simulink model "hydrothermal"  (R2018b)
settings: Solver=ode45  StartTime=0.0  StopTime=100  FixedStep=2  RelTol=1e-3
values from neighbouring files (symbols this model uses):
  optim_param = Best_pos    [main.m]
  w1 = 0.001    [main.m]
  w2 = 0.001    [main.m]
libraries: powerlib x1
settings Model: Creator=Orka  LastModifiedBy=Orka
settings SolverCC: ZeroCrossAlgorithm=Adaptive
settings DataIOCC: Refine=10
settings DebuggingCC: MaskedZcDiagnostic=none  IgnoredZcDiagnostic=none

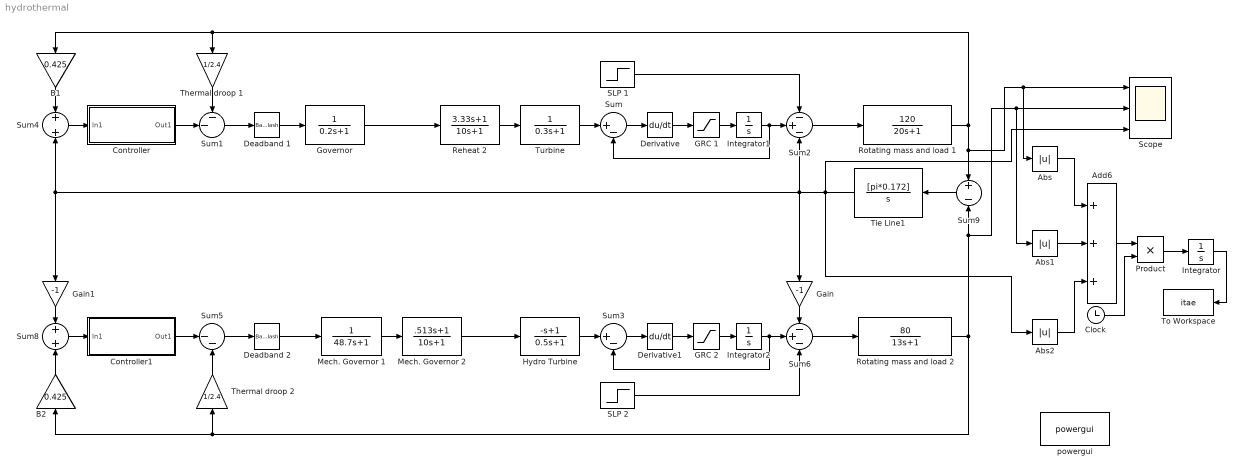
== system hydrothermal ==
  Abs : Abs
  Abs1 : Abs
  Abs2 : Abs
  Add6 : Sum  Inputs=+++
  B1 : Gain  Gain=0.425
  B2 : Gain  Gain=0.425
  Clock : Clock
  Controller : Subsystem
  Controller1 : Subsystem
  Deadband 1 : Backlash  BacklashWidth=0.0005
  Deadband 2 : Backlash  BacklashWidth=0.0002
  Derivative : Derivative
  Derivative1 : Derivative
  GRC 1 : Saturate  UpperLimit=0.0017  LowerLimit=-0.0017
  GRC 2 : Saturate  UpperLimit=0.045  LowerLimit=-0.06
  Gain : Gain  Gain=-1
  Gain1 : Gain  Gain=-1
  Governor : TransferFcn  Denominator=[0.2 1]
  Hydro Turbine : TransferFcn  Numerator=[-1 1]  Denominator=[0.5 1]
  Integrator : Integrator
  Integrator1 : Integrator
  Integrator2 : Integrator
  Mech. Governor 1 : TransferFcn  Denominator=[48.7 1]
  Mech. Governor 2 : TransferFcn  Numerator=[.513 1]  Denominator=[10 1]
  Product : Product
  Reheat 2 : TransferFcn  Numerator=[3.33 1]  Denominator=[10 1]
  Rotating mass and load 1 : TransferFcn  Numerator=[120]  Denominator=[20 1]
  Rotating mass and load 2 : TransferFcn  Numerator=[80]  Denominator=[13 1]
  SLP 1 : Step  After=w1  SampleTime=0
  SLP 2 : Step  After=w2  SampleTime=0
  Scope : Scope  NumInputPorts=3
  Sum : Sum  Inputs=|+-
  Sum1 : Sum  Inputs=--|
  Sum2 : Sum  Inputs=-+-
  Sum3 : Sum  Inputs=|+-
  Sum4 : Sum
  Sum5 : Sum  Inputs=|--
  Sum6 : Sum  Inputs=-+-
  Sum8 : Sum
  Sum9 : Sum  Inputs=+-
  Thermal droop 1 : Gain  Gain=1/2.4
  Thermal droop 2 : Gain  Gain=1/2.4
  Tie Line1 : TransferFcn  Numerator=[pi*0.172]  Denominator=[1 0]
  To Workspace : ToWorkspace  VariableName=itae  SampleTime=-1
  Turbine : TransferFcn  Denominator=[0.3 1]
  powergui : powerlib/powergui  Priority=1  SimulationMode=Discrete  SampleTime=50e-6  frequency=60  Iterations=50  frequencyindice=60  Pbase=100e6  ErrMax=1e-4  UnitsV=kV  UnitsW=MW  buscounter=0  FunctionMessages=off  echomessages=off  EnableUseOfTLC=off  CurrentSourceSwitches=off  DisableSnubberDevices=off  DisableRonSwitches=off  DisableVfSwitches=off  DisplayEquations=off  SolverType=Tustin/Backward Euler (TBE)  Interpol=off  ExternalGateDelay=off  methode=off  Ts=100  x0status=blocks  SPID=off  SwTol=0  HookPort=off  RestoreLinks=warning  ResistiveCurrentMeasurement=off  Frange=[0:2:500]  Ylog=off  Xlog=on  ShowGrid=off  save=off  variable=ZData  structure=0  ZoomFFT=off  StartTime=0.0  cycles=1  DisplayStyle=1  fundamental=60  FreqAxis=off  MaxFrequency=1000  frequencyindicesteady=1  RmsSteady=1  display=off
  wires:
  Rotating mass and load 2/1 -> Thermal droop 2/1, B2/1, Abs1/1, Scope/2, Sum9/2
  Integrator/1 -> To Workspace/1
  B2/1 -> Sum8/2
  Add6/1 -> Product/1
  Abs1/1 -> Add6/2
  Controller/1(Out1) -> Sum1/2
  Abs2/1 -> Add6/3
  Tie Line1/1 -> Abs2/1, Scope/3, Sum2/3, Gain/1, Gain1/1, Sum4/2
  Clock/1 -> Product/2
  Abs/1 -> Add6/1
  Product/1 -> Integrator/1
  Rotating mass and load 1/1 -> Abs/1, Scope/1, Sum9/1, B1/1, Thermal droop 1/1
  Sum8/1 -> Controller1/1(In1)
  Sum4/1 -> Controller/1(In1)
  Sum2/1 -> Rotating mass and load 1/1
  Thermal droop 1/1 -> Sum1/1
  SLP 1/1 -> Sum2/1
  Sum6/1 -> Rotating mass and load 2/1
  Sum9/1 -> Tie Line1/1
  B1/1 -> Sum4/1
  Controller1/1(Out1) -> Sum5/1
  Thermal droop 2/1 -> Sum5/2
  Governor/1 -> Reheat 2/1
  Reheat 2/1 -> Turbine/1
  SLP 2/1 -> Sum6/3
  Gain/1 -> Sum6/1
  Gain1/1 -> Sum8/1
  Mech. Governor 1/1 -> Mech. Governor 2/1
  Mech. Governor 2/1 -> Hydro Turbine/1
  Turbine/1 -> Sum/1
  Sum/1 -> Derivative/1
  Derivative/1 -> GRC 1/1
  GRC 1/1 -> Integrator1/1
  Integrator1/1 -> Sum/2, Sum2/2
  Integrator2/1 -> Sum6/2, Sum3/2
  Hydro Turbine/1 -> Sum3/1
  Derivative1/1 -> GRC 2/1
  GRC 2/1 -> Integrator2/1
  Sum3/1 -> Derivative1/1
  Deadband 1/1 -> Governor/1
  Sum1/1 -> Deadband 1/1
  Sum5/1 -> Deadband 2/1
  Deadband 2/1 -> Mech. Governor 1/1

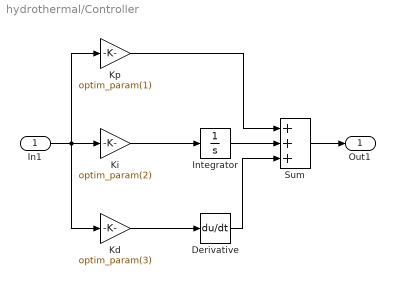
== system hydrothermal/Controller ==
  In1 : Inport
  Derivative : Derivative
  Integrator : Integrator
  Kd : Gain  Gain=optim_param(3)
  Ki : Gain  Gain=optim_param(2)
  Kp : Gain  Gain=optim_param(1)
  Sum : Sum  Inputs=+++
  Out1 : Outport
  wires:
  Sum/1 -> Out1/1
  Integrator/1 -> Sum/2
  Ki/1 -> Integrator/1
  Kd/1 -> Derivative/1
  Derivative/1 -> Sum/3
  In1/1 -> Kd/1, Kp/1, Ki/1
  Kp/1 -> Sum/1

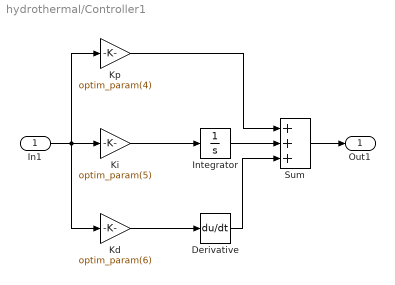
== system hydrothermal/Controller1 ==
  In1 : Inport
  Derivative : Derivative
  Integrator : Integrator
  Kd : Gain  Gain=optim_param(6)
  Ki : Gain  Gain=optim_param(5)
  Kp : Gain  Gain=optim_param(4)
  Sum : Sum  Inputs=+++
  Out1 : Outport
  wires:
  Sum/1 -> Out1/1
  Integrator/1 -> Sum/2
  Ki/1 -> Integrator/1
  Kd/1 -> Derivative/1
  Derivative/1 -> Sum/3
  In1/1 -> Kd/1, Kp/1, Ki/1
  Kp/1 -> Sum/1
